simulink model "ThdRwRtStCshnFldCtrl"  (R2024b)
settings: Solver=FixedStepDiscrete  StartTime=0.0  StopTime=10.0  FixedStep=0.01  RelTol=1e-3
undefined symbols (not defined in the file or in its folder): KeSMSuMdMotFinshdTm_Val, KeSMSuMdRetryTm1_Val, KeSMSuModeReqDurgTm_Val
libraries: StCtrlLib x1
settings Model: Creator=sn2xws  LastModifiedBy=sn55gm
settings SolverCC: AlgebraicLoopSolver=TrustRegion
settings DataIOCC: SaveFormat=StructureWithTime  ReturnWorkspaceOutputs=off
settings OptimizationCC: DefaultParameterBehavior=Inlined  EnhancedBackFolding=on  PassReuseOutputArgsAs=Individual arguments  ZeroExternalMemoryAtStartup=off  ZeroInternalMemoryAtStartup=off  OptimizeBlockOrder=speed  DifferentSizesBufferReuse=on  OptimizationCustomize=off  EfficientTunableParamExpr=on
settings DebuggingCC: ParameterTunabilityLossMsg=error  UnconnectedInputMsg=warning  UnconnectedOutputMsg=warning  UnconnectedLineMsg=warning  ArithmeticOperatorsInVariantConditions=warning
settings ModelReferenceCC: EnableRefExpFcnMdlSchedulingChecks=on  ModelReferenceNumInstancesAllowed=Single
settings SFSimCC: MATLABDynamicMemAlloc=off  CustomCodeUndefinedFunction=UseInterfaceOnly
settings RTWCC: Description=AUTOSAR  SystemTargetFile=autosar.tlc  GenCodeOnly=on  TemplateMakefile=ert_default_tmf  GenerateReport=on  IncludeHyperlinkInReport=on  LaunchReport=on  DataTypeReplacement=CDataTypesFixedWidth  GenerateTraceInfo=on  GenerateTraceReport=on  GenerateTraceReportSl=on  GenerateTraceReportSf=on  GenerateTraceReportEml=on  GPUComputeCapability=3.5
settings CodeAppCC: ForceParamTrailComments=on  IgnoreCustomStorageClasses=off  OperatorAnnotations=on  SimulinkDataObjDesc=on  SFDataObjDesc=on  InsertBlockDesc=on
settings STFCustomTargetCC: TargetLangStandard=C99 (ISO)  MultiwordLength=256  ParMdlRefBuildCompliant=on  CompOptLevelCompliant=on  IncludeMdlTerminateFcn=off  CombineOutputUpdateFcns=on  SuppressErrorStatus=on  ERTCustomFileBanners=on  SupportNonFinite=off  SupportComplex=off  SupportContinuousTime=off  SupportNonInlinedSFcns=off  RemoveResetFunc=on  MATLABClassNameForMDSCustomization=Simulink.SoftwareTarget.ERTCustomization  AutosarCompliant=on  UseToolchainInfoCompliant=on  LookupTableObjectStructAxisOrder=2,1,3,4,...  LUTObjectStructOrderEvenSpacing=Size,Table,Breakpoints  SystemTargetFile=autosar.tlc
settings ERTTargetCC: TargetLangStandard=C99 (ISO)  ConcurrentExecutionCompliant=off  IncludeMdlTerminateFcn=off  SuppressErrorStatus=on  SupportNonFinite=off  SupportComplex=off  ModelStepFunctionPrototypeControlCompliant=off  CPPClassGenCompliant=off  AutosarCompliant=on  LookupTableObjectStructAxisOrder=2,1,3,4,...  LUTObjectStructOrderEvenSpacing=Size,Table,Breakpoints  ERTCustomFileTemplate=example_file_process.tlc  ERTFilePackagingFormat=Compact  BooleanTrueId=TRUE  BooleanFalseId=FALSE  DynamicArrayContainerType=coder::array

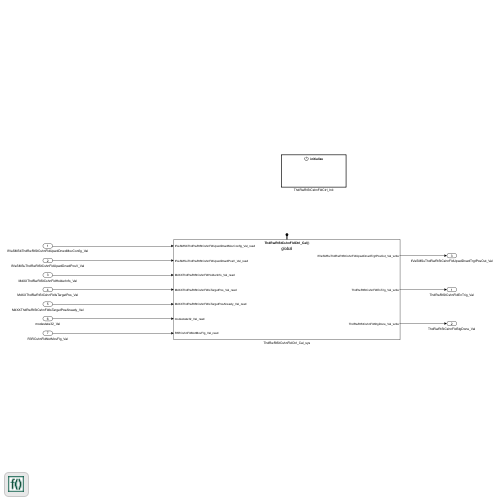
[thumbnail: Simulink's stored preview of the top-level diagram]
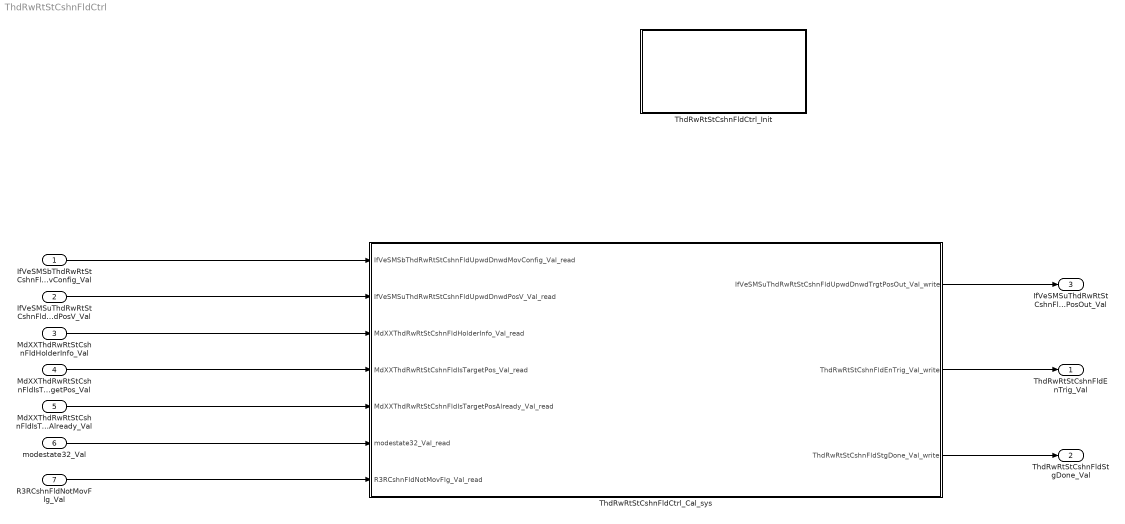
== system ThdRwRtStCshnFldCtrl ==
  IfVeSMSbThdRwRtStCshnFldUpwdDnwdMovConfig_Val : Inport  OutDataTypeStr=boolean  PortDimensions=1
  IfVeSMSuThdRwRtStCshnFldUpwdDnwdPosV_Val : Inport  Port=2  OutDataTypeStr=boolean  PortDimensions=1
  MdXXThdRwRtStCshnFldHolderInfo_Val : Inport  Port=3  OutDataTypeStr=uint32  PortDimensions=1
  MdXXThdRwRtStCshnFldIsTargetPos_Val : Inport  Port=4  OutDataTypeStr=uint32  PortDimensions=1
  MdXXThdRwRtStCshnFldIsTargetPosAlready_Val : Inport  Port=5  OutDataTypeStr=uint32  PortDimensions=1
  modestate32_Val : Inport  Port=6  OutDataTypeStr=uint32  PortDimensions=1
  R3RCshnFldNotMovFlg_Val : Inport  Port=7  OutDataTypeStr=boolean  PortDimensions=1
  ThdRwRtStCshnFldCtrl_Cal_sys : Subsystem
  ThdRwRtStCshnFldCtrl_Init : Subsystem
  ThdRwRtStCshnFldEnTrig_Val : Outport  OutDataTypeStr=boolean  PortDimensions=1  VectorParamsAs1DForOutWhenUnconnected=off
  ThdRwRtStCshnFldStgDone_Val : Outport  Port=2  OutDataTypeStr=boolean  PortDimensions=1  VectorParamsAs1DForOutWhenUnconnected=off
  IfVeSMSuThdRwRtStCshnFldUpwdDnwdTrgtPosOut_Val : Outport  Port=3  OutDataTypeStr=boolean  PortDimensions=1  VectorParamsAs1DForOutWhenUnconnected=off
  wires:
  IfVeSMSbThdRwRtStCshnFldUpwdDnwdMovConfig_Val/1 -> ThdRwRtStCshnFldCtrl_Cal_sys/1(IfVeSMSbThdRwRtStCshnFldUpwdDnwdMovConfig_Val_read)
  IfVeSMSuThdRwRtStCshnFldUpwdDnwdPosV_Val/1 -> ThdRwRtStCshnFldCtrl_Cal_sys/2(IfVeSMSuThdRwRtStCshnFldUpwdDnwdPosV_Val_read)
  MdXXThdRwRtStCshnFldHolderInfo_Val/1 -> ThdRwRtStCshnFldCtrl_Cal_sys/3(MdXXThdRwRtStCshnFldHolderInfo_Val_read)
  MdXXThdRwRtStCshnFldIsTargetPos_Val/1 -> ThdRwRtStCshnFldCtrl_Cal_sys/4(MdXXThdRwRtStCshnFldIsTargetPos_Val_read)
  MdXXThdRwRtStCshnFldIsTargetPosAlready_Val/1 -> ThdRwRtStCshnFldCtrl_Cal_sys/5(MdXXThdRwRtStCshnFldIsTargetPosAlready_Val_read)
  modestate32_Val/1 -> ThdRwRtStCshnFldCtrl_Cal_sys/6(modestate32_Val_read)
  R3RCshnFldNotMovFlg_Val/1 -> ThdRwRtStCshnFldCtrl_Cal_sys/7(R3RCshnFldNotMovFlg_Val_read)
  ThdRwRtStCshnFldCtrl_Cal_sys/1(IfVeSMSuThdRwRtStCshnFldUpwdDnwdTrgtPosOut_Val_write) -> IfVeSMSuThdRwRtStCshnFldUpwdDnwdTrgtPosOut_Val/1
  ThdRwRtStCshnFldCtrl_Cal_sys/2(ThdRwRtStCshnFldEnTrig_Val_write) -> ThdRwRtStCshnFldEnTrig_Val/1
  ThdRwRtStCshnFldCtrl_Cal_sys/3(ThdRwRtStCshnFldStgDone_Val_write) -> ThdRwRtStCshnFldStgDone_Val/1

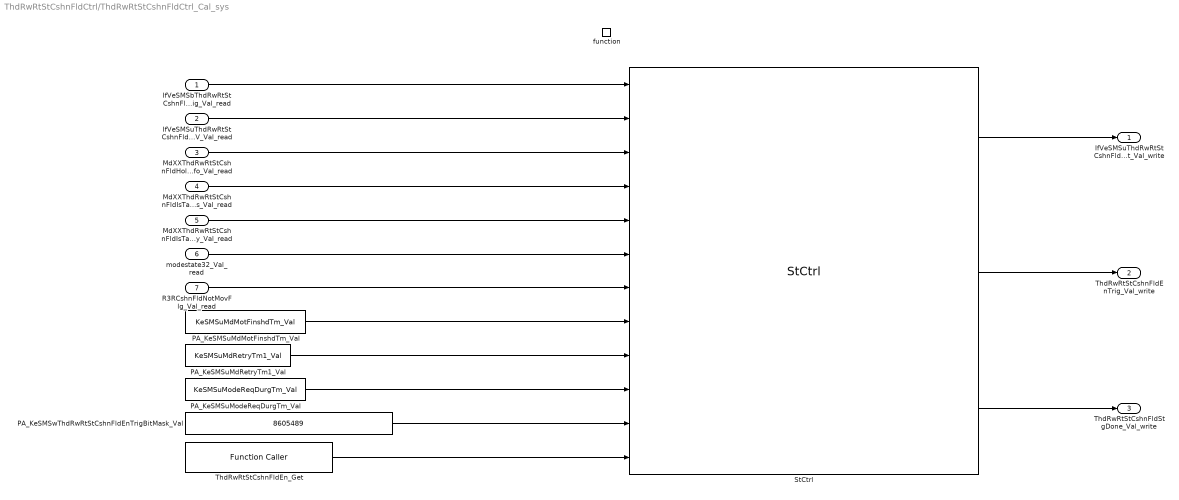
== system ThdRwRtStCshnFldCtrl/ThdRwRtStCshnFldCtrl_Cal_sys ==
  IfVeSMSbThdRwRtStCshnFldUpwdDnwdMovConfig_Val_read : Inport
  IfVeSMSuThdRwRtStCshnFldUpwdDnwdPosV_Val_read : Inport  Port=2
  MdXXThdRwRtStCshnFldHolderInfo_Val_read : Inport  Port=3
  MdXXThdRwRtStCshnFldIsTargetPos_Val_read : Inport  Port=4
  MdXXThdRwRtStCshnFldIsTargetPosAlready_Val_read : Inport  Port=5
  modestate32_Val_read : Inport  Port=6
  R3RCshnFldNotMovFlg_Val_read : Inport  Port=7
  function : TriggerPort  TriggerType=function-call  IsSimulinkFunction=on  FunctionName=ThdRwRtStCshnFldCtrl_Cal  VariantControl=(inherit)
  PA_KeSMSuMdMotFinshdTm_Val : Constant  Value=KeSMSuMdMotFinshdTm_Val
  PA_KeSMSuMdRetryTm1_Val : Constant  Value=KeSMSuMdRetryTm1_Val
  PA_KeSMSuModeReqDurgTm_Val : Constant  Value=KeSMSuModeReqDurgTm_Val
  PA_KeSMSwThdRwRtStCshnFldEnTrigBitMask_Val : Constant  Value=8605489  OutDataTypeStr=uint32
  StCtrl : StCtrlLib/StCtrl  SystemSampleTime=-1  VariantActivationTime=update diagram  AllowFlexibleInterface=on  Latency=0  AutoFrameSizeCalculation=off
  ThdRwRtStCshnFldEn_Get : FunctionCaller  FunctionPrototype=data = ThdRwRtStCshnFldEn_Get()  InputArgumentSpecifications=<Enter example>  OutputArgumentSpecifications=uint32(1)
  IfVeSMSuThdRwRtStCshnFldUpwdDnwdTrgtPosOut_Val_write : Outport  VectorParamsAs1DForOutWhenUnconnected=off
      settings: EnsureOutportIsVirtual=on
  ThdRwRtStCshnFldEnTrig_Val_write : Outport  Port=2  VectorParamsAs1DForOutWhenUnconnected=off
      settings: EnsureOutportIsVirtual=on
  ThdRwRtStCshnFldStgDone_Val_write : Outport  Port=3  VectorParamsAs1DForOutWhenUnconnected=off
      settings: EnsureOutportIsVirtual=on
  wires:
  StCtrl/1 -> IfVeSMSuThdRwRtStCshnFldUpwdDnwdTrgtPosOut_Val_write/1
  StCtrl/2 -> ThdRwRtStCshnFldEnTrig_Val_write/1
  StCtrl/3 -> ThdRwRtStCshnFldStgDone_Val_write/1
  PA_KeSMSwThdRwRtStCshnFldEnTrigBitMask_Val/1 -> StCtrl/11
  ThdRwRtStCshnFldEn_Get/1 -> StCtrl/12
  PA_KeSMSuMdMotFinshdTm_Val/1 -> StCtrl/8
  PA_KeSMSuModeReqDurgTm_Val/1 -> StCtrl/10
  PA_KeSMSuMdRetryTm1_Val/1 -> StCtrl/9
  MdXXThdRwRtStCshnFldHolderInfo_Val_read/1 -> StCtrl/3
  IfVeSMSuThdRwRtStCshnFldUpwdDnwdPosV_Val_read/1 -> StCtrl/2
  IfVeSMSbThdRwRtStCshnFldUpwdDnwdMovConfig_Val_read/1 -> StCtrl/1
  MdXXThdRwRtStCshnFldIsTargetPos_Val_read/1 -> StCtrl/4
  MdXXThdRwRtStCshnFldIsTargetPosAlready_Val_read/1 -> StCtrl/5
  modestate32_Val_read/1 -> StCtrl/6
  R3RCshnFldNotMovFlg_Val_read/1 -> StCtrl/7

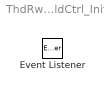
== system ThdRwRtStCshnFldCtrl/ThdRwRtStCshnFldCtrl_Init ==
  Event Listener : EventListener  EventName=reset
